simulink model "transferFunction"  (R2023b)
settings: Solver=VariableStepAuto  StartTime=0.0  StopTime=10.0  RelTol=1e-3
libraries: simulink x1

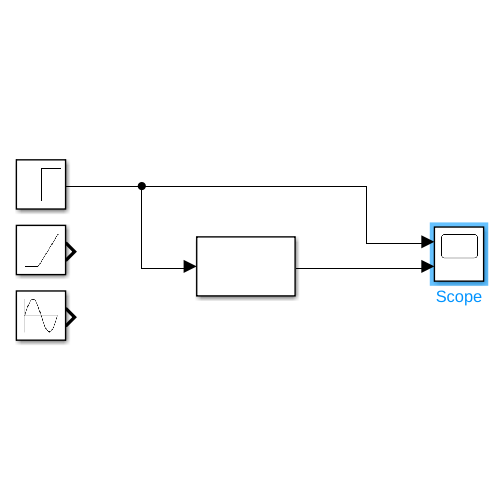
[thumbnail: Simulink's stored preview of the top-level diagram]
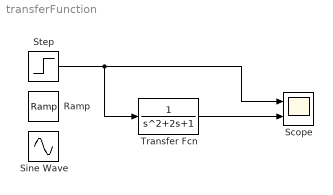
== system transferFunction ==
  Ramp : simulink/Sources/Ramp  slope=1  start=0  InitialOutput=0
  Scope : Scope  NumInputPorts=2
  Sine Wave : Sin  SampleTime=0
  Step : Step  SampleTime=0
  Transfer Fcn : TransferFcn
  wires:
  Transfer Fcn/1 -> Scope/2
  Step/1 -> Transfer Fcn/1, Scope/1
